simulink model "craneGA"  (R2023b)
settings: Solver=VariableStepAuto  StartTime=0.0  StopTime=sim_time  FixedStep=sim_step  MaxStep=sim_step  RelTol=1e-3
values from neighbouring files (symbols this model uses):
  C = Pop(i,3)    [GA.m]    (also in izka.mat = 4.74862786183; meranie1.mat = 11.3345130893; meranie2.mat = 10.8395112259; meranie3.mat = 10.5647928076)
  F_cart_den = [2.813749053553513e-05	1	0]    [GA.m]    (also in izka.mat = [2.81374905355e-05 1 0]; meranie1.mat = [2.81374905355e-05 1 0]; meranie2.mat = [2.81374905355e-05 1 0]; meranie3.mat = [2.81374905355e-05 1 0])
  F_cart_num = [0	0	0.217598139970441]    [GA.m]    (also in izka.mat = [0 0 0.21759813997]; meranie1.mat = [0 0 0.21759813997]; meranie2.mat = [0 0 0.21759813997]; meranie3.mat = [0 0 0.21759813997])
  F_pend_den = [1	0.0125366535496897	12.9568004970019]    [GA.m]    (also in izka.mat = [1 0.0125366535497 12.956800497]; meranie1.mat = [1 0.0125366535497 12.956800497]; meranie2.mat = [1 0.0125366535497 12.956800497]; meranie3.mat = [1 0.0125366535497 12.956800497])
  F_pend_num = [-1.37069413493978	0	0]    [GA.m]    (also in izka.mat = [-1.37069413494 0 0]; meranie1.mat = [-1.37069413494 0 0]; meranie2.mat = [-1.37069413494 0 0]; meranie3.mat = [-1.37069413494 0 0])
  I = Pop(i,2)    [GA.m]    (also in izka.mat = 7.78140484293; meranie1.mat = 0.526099986265; meranie2.mat = 3.05318784953; meranie3.mat = 0.594304323923)
  P = Pop(i,1)    [GA.m]    (also in izka.mat = 9.77813174253; meranie1.mat = 6.16880734651; meranie2.mat = 6.25392782724; meranie3.mat = 8.1585790558)
libraries: slpidlib x1, SignalEditorBlockLib x1
settings Model: Creator=maros-pc  LastModifiedBy=maros-pc
settings SolverCC: EnableFixedStepZeroCrossing=on  MaxZcPerStep=5

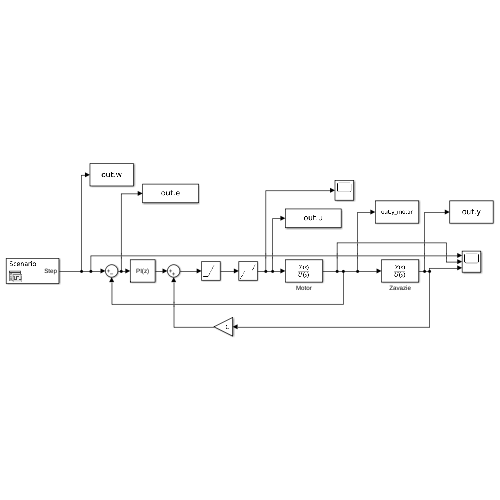
[thumbnail: Simulink's stored preview of the top-level diagram]
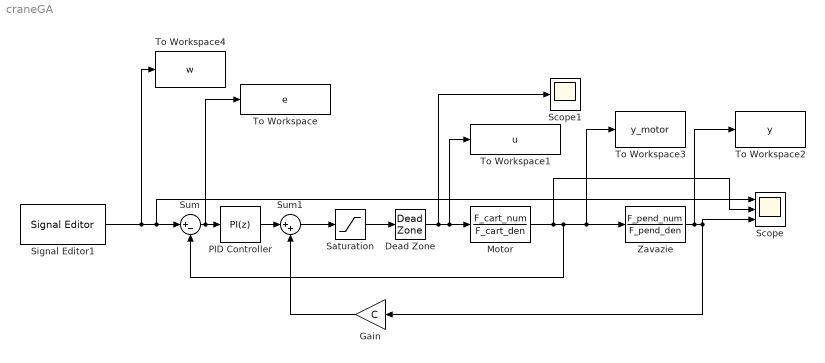
== system craneGA ==
  Dead Zone : DeadZone  LowerValue=-0.2  UpperValue=0.2
  Gain : Gain  Gain=C
  Motor : TransferFcn  Numerator=F_cart_num  Denominator=F_cart_den
  PID Controller : slpidlib/PID Controller  Controller=PI  Form=Parallel  TimeDomain=Discrete-time  UseExternalTs=off  SampleTime=-1  IntegratorMethod=Forward Euler  FilterMethod=Forward Euler  ControllerParametersSource=internal  P=P  I=I  UseKiTs=off  D=0  N=100  UseFilter=on  TunerSelectOption=Transfer Function Based (PID Tuner App)  InitialConditionSource=internal  InitialConditionForIntegrator=0  InitialConditionForFilter=0  DifferentiatorICPrevScaledInput=0  ExternalReset=none  TrackingMode=off  Kt=1  LimitOutput=off  SatLimitsSource=internal  UpperSaturationLimit=inf  LowerSaturationLimit=-inf  LinearizeAsGain=on  AntiWindupMode=none  Kb=1  LimitIntegrator=off  UpperIntegratorSaturationLimit=inf  LowerIntegratorSaturationLimit=-inf  POutMin=[]  POutMax=[]  IOutMin=[]  IOutMax=[]  DOutMin=[]  DOutMax=[]  NOutMin=[]  NOutMax=[]  SumOutMin=[]  SumOutMax=[]  SaturationOutMin=[]  SaturationOutMax=[]  PParamMin=[]  PParamMax=[]  IParamMin=[]  IParamMax=[]  DParamMin=[]  DParamMax=[]  NParamMin=[]  NParamMax=[]  KbParamMin=[]  KbParamMax=[]  KtParamMin=[]  KtParamMax=[]  KbOutMin=[]  KbOutMax=[]  KtOutMin=[]  KtOutMax=[]  IntegratorOutMin=[]  IntegratorOutMax=[]  FilterOutMin=[]  FilterOutMax=[]  SumI1OutMin=[]  SumI1OutMax=[]  SumI2OutMin=[]  SumI2OutMax=[]  SumI3OutMin=[]  SumI3OutMax=[]  SumI4OutMin=[]  SumI4OutMax=[]  SumDOutMin=[]  SumDOutMax=[]  DifferentiatorOutMin=[]  DifferentiatorOutMax=[]  FilterDiffOutCoefMin=[]  FilterDiffOutCoefMax=[]  ReciprocalOutMin=[]  ReciprocalOutMax=[]  SumDenOutMin=[]  SumDenOutMax=[]  SumNumOutMin=[]  SumNumOutMax=[]  DivideOutMin=[]  DivideOutMax=[]  UdiffTsProdOutMin=[]  UdiffTsProdOutMax=[]  NTsProdOutMin=[]  NTsProdOutMax=[]  UintegralTsProdOutMin=[]  UintegralTsProdOutMax=[]  UngainTsProdOutMin=[]  UngainTsProdOutMax=[]  ClampingZeroOutDataTypeStr=Inherit: Inherit via back propagation  ClampingZeroOutMin=[]  ClampingZeroOutMax=[]  FilterDenConstantOutDataTypeStr=Inherit: Inherit via back propagation  FilterDenConstantOutMin=[]  FilterDenConstantOutMax=[]  PCopyOutDataTypeStr=Inherit: Inherit via back propagation  PCopyOutMin=[]  PCopyOutMax=[]  NCopyOutDataTypeStr=Inherit: Inherit via back propagation  NCopyOutMin=[]  NCopyOutMax=[]  IntegratorContinuousStateAttributes=''  IntegratorStateMustResolveToSignalObject=off  IntegratorRTWStateStorageClass=Auto  FilterContinuousStateAttributes=''  FilterStateMustResolveToSignalObject=off  FilterRTWStateStorageClass=Auto  ParallelPVariant=InternalParameters  IdealPVariant=Disabled  IVariant=InternalParameters  DVariant=Disabled  IntegratorVariant=Discrete  SatVariant=Disabled  AWVariant=Passthrough  PCopyVariant=Disabled  TRVariant=Disabled  FdbkBlocksVariant=Forward  IdealPFdbkVariant=Disabled  SatFdbkVariant=Disabled  DerivativeFilterVariant=Disabled  NVariant=Disabled  NCopyVariant=Disabled_SignalSpec  FilterICVariant=Disabled  IntegratorICVariant=InternalICs  ExternalResetVariant=Disabled  TRSumVariant=Passthrough  SumFdbkVariant=Disabled  SumVariant=Sum_PI  TsampFilterVariant=InternalTs  TsampNgainVariant=Passthrough  TsampIntegralVariant=Disabled_SignalSpec  ExternalSaturationOutDataTypeStr=Inherit: Same as second input
  Saturation : Saturate  UpperLimit=1  LowerLimit=-1
  Scope : Scope  NumInputPorts=3
  Scope1 : Scope
  Signal Editor1 : SignalEditorBlockLib/Signal Editor  FileName=ziadana_polohax.mat  ActiveScenario=Scenario  ActiveSignal=Step  IsBus=off  OutputBusObjectStr=Bus: BusObject  SampleTime=0  Interpolate=off  ZeroCross=off  OutputAfterFinalValue=Setting to zero  Unit=inherit  PreserveSignalName=on  ApplySigPropsToAllScenarios=on  ApplySigPropsToAllSignals=off
  Sum : Sum  Inputs=|+-
  Sum1 : Sum  Inputs=|++
  To Workspace : ToWorkspace  VariableName=e  SaveFormat=Timeseries  SampleTime=-1
  To Workspace1 : ToWorkspace  VariableName=u  SaveFormat=Timeseries  SampleTime=-1
  To Workspace2 : ToWorkspace  VariableName=y  SaveFormat=Timeseries  SampleTime=-1
  To Workspace3 : ToWorkspace  VariableName=y_motor  SaveFormat=Timeseries  SampleTime=-1
  To Workspace4 : ToWorkspace  VariableName=w  SaveFormat=Timeseries  SampleTime=-1
  Zavazie : TransferFcn  Numerator=F_pend_num  Denominator=F_pend_den
  wires:
  Zavazie/1 -> To Workspace2/1, Gain/1, Scope/3
  Motor/1 -> Scope/2, Sum/2, To Workspace3/1, Zavazie/1
  Sum/1 -> To Workspace/1, PID Controller/1
  Gain/1 -> Sum1/2
  Sum1/1 -> Saturation/1
  Saturation/1 -> Dead Zone/1
  Dead Zone/1 -> Scope1/1, To Workspace1/1, Motor/1
  PID Controller/1 -> Sum1/1
  Signal Editor1/1 -> To Workspace4/1, Scope/1, Sum/1
